simulink model "cyclic_prefix_of_4_symbol"  (R2022a)
settings: Solver=VariableStepAuto  StartTime=0.0  StopTime=5000  RelTol=1e-3
undefined symbols (not defined in the file): xc7s100fgga676
libraries: hdlBasic x19, commrandsrc3 x1, commsink2 x1, vmcUtilities x1
settings Model: Creator=Sandesh  LastModifiedBy=Sandesh

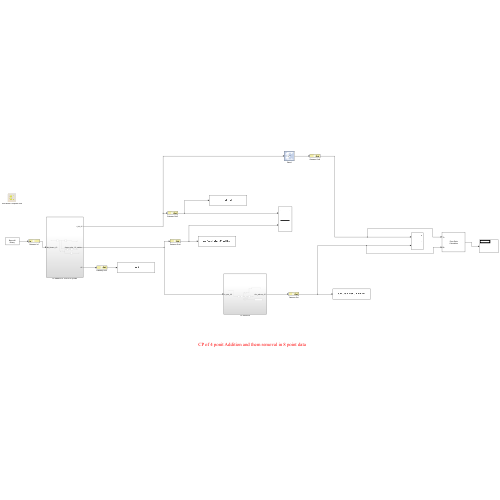
[thumbnail: Simulink's stored preview of the top-level diagram]
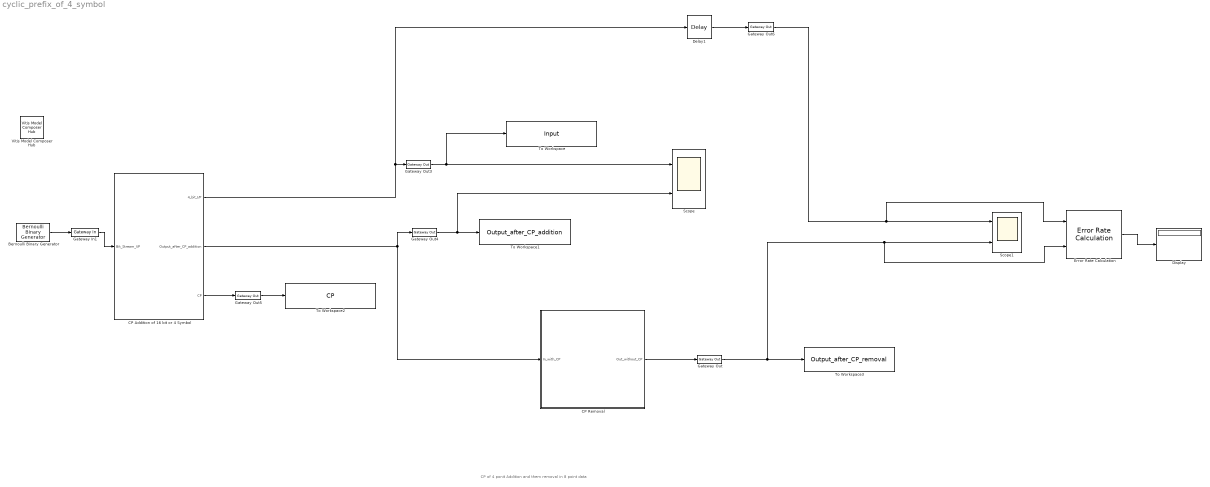
== system cyclic_prefix_of_4_symbol ==
  note: CP of 4 ponit Addition and them removal in 8 point data
  Bernoulli Binary Generator : commrandsrc3/Bernoulli Binary Generator  ProbabilityOfZero=0.5  SeedSource=Auto  Seed=0  SampleTime=1  SamplesPerFrame=1  OutputDataType=double  SimulateUsing=Interpreted execution
  CP Addition of 16 bit or 4 Symbol : Subsystem
  CP Removal : Subsystem
  Delay1 : hdlBasic/Delay  rst=off  en=off  latency=16  reg_retiming=off  XmcBlockStatus=1  maskContainerNames=group1  block_type=delay  block_config=sysgen:Delay_config
  Display : Display
  Error Rate Calculation : commsink2/Error Rate Calculation  N=0  st_delay=0  cp_mode=Entire frame  subframe=[]  PMode=Port  WsName=ErrorVec  RsMode2=off  stop=off  numErr=100  maxBits=1e6
  Gateway In1 : hdlBasic/Gateway In  gui_display_data_type=Fixed-point  arith_type=Unsigned  n_bits=1  bin_pt=0  preci_type=Single  exp_width=8  frac_width=24  rows=1  columns=1  quantization="Round  (unbiased: +/- Inf)"  overflow=Saturate  period=1  UseAsADC=off  ADCChannel='1'  interface=None  automatic_assignment=on  address_offset=hex2dec('00')  intf_name=''  intf_description=''  default_value=0  timing_constraint=None  locs_specified=off  LOCs={}  io_standard={}  inherit_from_input=off  hdl_port=on  XmcBlockStatus=1  maskContainerNames=group4  block_type=gatewayin  block_config=sysgen:gateway_in_config  block_width_w=590  block_height_w=620  block_width=640  block_height=850
  Gateway Out{,3..6} (5 alike) : hdlBasic/Gateway Out  inherit_from_input=off  hdl_port=on  rows=1  columns=1  UseAsDAC=off  DACChannel='1'  interface=None  automatic_assignment=on  address_offset=hex2dec('00')  intf_name=''  intf_description=''  timing_constraint=None  locs_specified=off  LOCs={}  io_standard={}  XmcBlockStatus=1  maskContainerNames=group4  block_type=gatewayout  block_config=sysgen:gateway_out_config  block_width_w=590  block_height_w=620  block_width=620  block_height=750
  Scope : Scope  NumInputPorts=2
  Scope1 : Scope  NumInputPorts=2
  To Workspace : ToWorkspace  VariableName=Input  SaveFormat=Timeseries  SampleTime=-1
  To Workspace1 : ToWorkspace  VariableName=Output_after_CP_addition  SaveFormat=Timeseries  SampleTime=-1
  To Workspace2 : ToWorkspace  VariableName=CP  SaveFormat=Timeseries  SampleTime=-1
  To Workspace3 : ToWorkspace  VariableName=Output_after_CP_removal  SaveFormat=Timeseries  SampleTime=-1
  Vitis Model Composer Hub : vmcUtilities/Vitis Model Composer Hub  Tag=genX  CodeGeneration=off  TargetDirectory=./code  ExportType=AI Engines  IpVendor=xilinx.com  IpLibrary=hls  IpVersion=1.0  IpHWLanguage=Verilog  AieCompilerOptions={}  CreateTestbench=off  TestbenchStackSize=10  RunAieSim=off  AieSimTimeout=50000  RunAieSimProfiling=off  LaunchVitisAnalyzer=off  PlotOutput=off  RunX86Sim=off  X86SimTimeout=10  GenHwImage=off  PlatformType=Not Specified  HwSystemType=Baremetal  HwValidationTarget=hw  ProjDevice=Spartan-7 SP701 Evaluation Platform (xc7s100fgga676-2)  ProjDevicePart=xc7s100fgga676-2  SamplePeriod=-1  ClockFrequency=200  DataPathParallelism=1  xilinxfamily=spartan7  part=xc7s100  speed=-2  package=fgga676  directory=./netlist  testbench=off  incr_netlist=off  synthesis_tool=Vivado  clock_wrapper=Clock Enables  dbl_ovrd=According to Block Masks  dcm_input_clock_period=10  sysclk_period=10  simulink_period=1/3  eval_field=0
  wires:
  Gateway Out3/1 -> To Workspace/1, Scope/1
  Gateway Out4/1 -> Scope/2, To Workspace1/1
  Gateway Out5/1 -> To Workspace2/1
  Gateway Out/1 -> Error Rate Calculation/2, Scope1/2, To Workspace3/1
  Bernoulli Binary Generator/1 -> Gateway In1/1
  Gateway In1/1 -> CP Addition of 16 bit or 4 Symbol/1(Bit_Stream_I/P)
  CP Addition of 16 bit or 4 Symbol/1(4_bit_I/P) -> Delay1/1, Gateway Out3/1
  CP Addition of 16 bit or 4 Symbol/3(CP) -> Gateway Out5/1
  CP Addition of 16 bit or 4 Symbol/2(Output_after_CP_addition) -> Gateway Out4/1, CP Removal/1(In_with_CP)
  Delay1/1 -> Gateway Out6/1
  CP Removal/1(Out_without_CP) -> Gateway Out/1
  Gateway Out6/1 -> Error Rate Calculation/1, Scope1/1
  Error Rate Calculation/1 -> Display/1

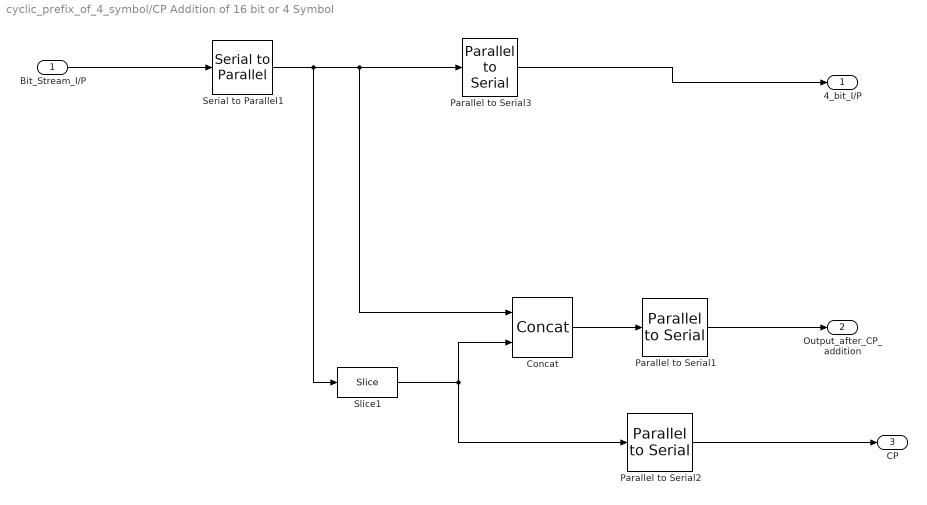
== system cyclic_prefix_of_4_symbol/CP Addition of 16 bit or 4 Symbol ==
  Bit_Stream_I/P : Inport
  Concat : hdlBasic/Concat  num_inputs=2  XmcBlockStatus=1  maskContainerNames=group1  block_type=concat  block_config=sysgen:Concat_config
  Parallel to Serial1 : hdlBasic/Parallel to Serial  output_order=Least Significant Word First  arith_type=Unsigned  output_bits=4  bin_pt=0  rst=off  en=off  latency=1  XmcBlockStatus=1  maskContainerNames=group1  block_type=p2s  block_config=sysgen:P2S_config
  Parallel to Serial2 : hdlBasic/Parallel to Serial  output_order=Least Significant Word First  arith_type=Unsigned  output_bits=4  bin_pt=0  rst=off  en=off  latency=1  XmcBlockStatus=1  maskContainerNames=group1  block_type=p2s  block_config=sysgen:P2S_config
  Parallel to Serial3 : hdlBasic/Parallel to Serial  output_order=Least Significant Word First  arith_type=Unsigned  output_bits=4  bin_pt=0  rst=off  en=off  latency=1  XmcBlockStatus=1  maskContainerNames=group1  block_type=p2s  block_config=sysgen:P2S_config
  Serial to Parallel1 : hdlBasic/Serial to Parallel  input_order=Least Significant Word First  arith_type=Unsigned  output_bits=32  bin_pt=0  rst=off  en=off  latency=1  input_bits=[]  XmcBlockStatus=1  maskContainerNames=group3  block_type=s2p  block_config=sysgen:S2P_config
  Slice1 : hdlBasic/Slice  nbits=16  boolean_output=off  mode=Upper Bit Location + Width  bit1=0  base1=MSB of Input  bit0=0  base0=LSB of Input  XmcBlockStatus=1  maskContainerNames=group1  block_type=slice  block_config=sysgen:Slice_config
  4_bit_I/P : Outport
  Output_after_CP_addition : Outport  Port=2
  CP : Outport  Port=3
  wires:
  Serial to Parallel1/1 -> Parallel to Serial3/1, Concat/1, Slice1/1
  Concat/1 -> Parallel to Serial1/1
  Slice1/1 -> Parallel to Serial2/1, Concat/2
  Bit_Stream_I/P/1 -> Serial to Parallel1/1
  Parallel to Serial1/1 -> Output_after_CP_addition/1
  Parallel to Serial3/1 -> 4_bit_I/P/1
  Parallel to Serial2/1 -> CP/1

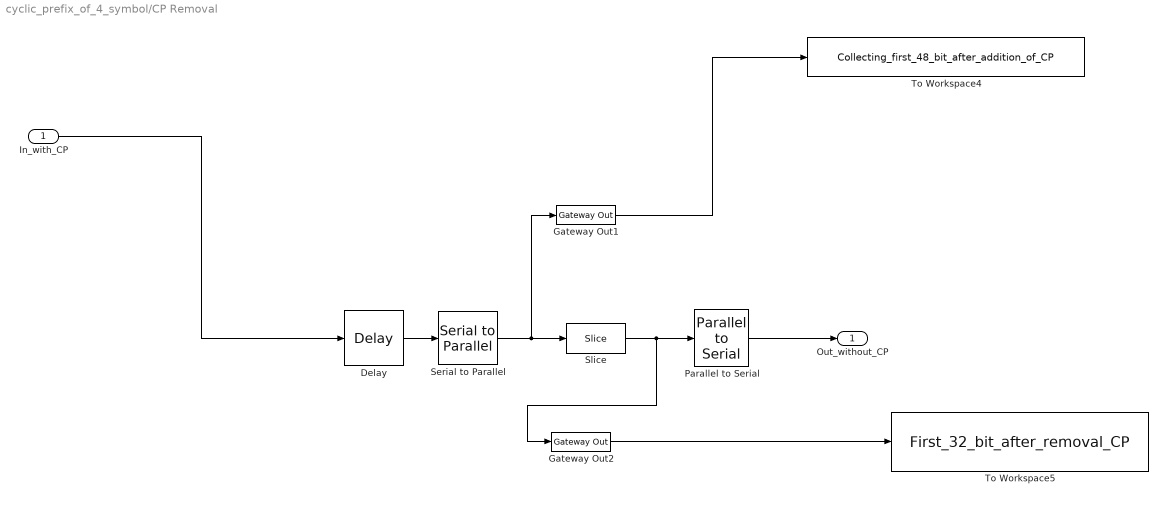
== system cyclic_prefix_of_4_symbol/CP Removal ==
  In_with_CP : Inport
  Delay : hdlBasic/Delay  rst=off  en=off  latency=11  reg_retiming=off  XmcBlockStatus=1  maskContainerNames=group1  block_type=delay  block_config=sysgen:Delay_config
  Gateway Out1 : hdlBasic/Gateway Out  inherit_from_input=off  hdl_port=on  rows=1  columns=1  UseAsDAC=off  DACChannel='1'  interface=None  automatic_assignment=on  address_offset=hex2dec('00')  intf_name=''  intf_description=''  timing_constraint=None  locs_specified=off  LOCs={}  io_standard={}  XmcBlockStatus=1  maskContainerNames=group4  block_type=gatewayout  block_config=sysgen:gateway_out_config  block_width_w=590  block_height_w=620  block_width=620  block_height=750
  Gateway Out2 : hdlBasic/Gateway Out  inherit_from_input=off  hdl_port=on  rows=1  columns=1  UseAsDAC=off  DACChannel='1'  interface=None  automatic_assignment=on  address_offset=hex2dec('00')  intf_name=''  intf_description=''  timing_constraint=None  locs_specified=off  LOCs={}  io_standard={}  XmcBlockStatus=1  maskContainerNames=group4  block_type=gatewayout  block_config=sysgen:gateway_out_config  block_width_w=590  block_height_w=620  block_width=620  block_height=750
  Parallel to Serial : hdlBasic/Parallel to Serial  output_order=Least Significant Word First  arith_type=Unsigned  output_bits=4  bin_pt=0  rst=off  en=off  latency=1  XmcBlockStatus=1  maskContainerNames=group1  block_type=p2s  block_config=sysgen:P2S_config
  Serial to Parallel : hdlBasic/Serial to Parallel  input_order=Least Significant Word First  arith_type=Unsigned  output_bits=48  bin_pt=0  rst=off  en=off  latency=1  input_bits=[]  XmcBlockStatus=1  maskContainerNames=group3  block_type=s2p  block_config=sysgen:S2P_config
  Slice : hdlBasic/Slice  nbits=32  boolean_output=off  mode=Upper Bit Location + Width  bit1=0  base1=MSB of Input  bit0=16  base0=LSB of Input  XmcBlockStatus=1  maskContainerNames=group1  block_type=slice  block_config=sysgen:Slice_config
  To Workspace4 : ToWorkspace  VariableName=Collecting_first_48_bit_after_addition_of_CP  SaveFormat=Timeseries  SampleTime=-1
  To Workspace5 : ToWorkspace  VariableName=First_32_bit_after_removal_CP  SaveFormat=Timeseries  SampleTime=-1
  Out_without_CP : Outport
  wires:
  Parallel to Serial/1 -> Out_without_CP/1
  Slice/1 -> Gateway Out2/1, Parallel to Serial/1
  Serial to Parallel/1 -> Gateway Out1/1, Slice/1
  In_with_CP/1 -> Delay/1
  Gateway Out1/1 -> To Workspace4/1
  Gateway Out2/1 -> To Workspace5/1
  Delay/1 -> Serial to Parallel/1
